simulink model "flexpes_phctrlr_sys"  (R2025b)
settings: Solver=VariableStepAuto  StartTime=0.0  StopTime=1e-6  RelTol=1e-3
values from neighbouring files (symbols this model uses):
  debouncer_cycles = 5    [choPLL_loop_impl.m]
  F_lock_thr = 1    [choPLL_loop_impl.m]
  FPGA_CLK = 125e6    (= 125000000)    [choPLL_loop_impl.m]
  FPGA_Ts = 1./FPGA_CLK    (= 8e-09)    [choPLL_loop_impl.m]
  IIR_C_X = G_loopfilt*my_num_loop_filtZ(1)    [choPLL_loop_impl.m]
  IIR_C_X1 = G_loopfilt*my_num_loop_filtZ(2)    [choPLL_loop_impl.m]
  IIR_C_Y1 = -my_den_loop_filtZ(2)    [choPLL_loop_impl.m]
  max_unwrap_periods = 50    [choPLL_loop_impl.m]
  PFD_CLK = 100e3    (= 100000)    [choPLL_loop_impl.m]
  PFD_Ts = 1./PFD_CLK    (= 1e-05)    [choPLL_loop_impl.m]
  PH_lock_thr = 4    [choPLL_loop_impl.m]
  PHCTRLR_CLK = 100    [choPLL_loop_impl.m]
  PHCTRLR_Ts = 1./PHCTRLR_CLK    (= 0.01)    [choPLL_loop_impl.m]
  TDC_cnt_per_period = round(FPGA_CLK/Fref)    [choPLL_loop_impl.m]
  unwrap_res_period_thr = 0    [choPLL_loop_impl.m]
  unwrap_reset_inhibit_cycles = 20000    [choPLL_loop_impl.m]
  wrap_detect_thr = round(TDC_cnt_per_period*0.55)    [choPLL_loop_impl.m]
libraries: hdlBasic x276, hdlUtilities x4, hdlDSPIP x4, vmcUtilities x1
(part 3 of 3)

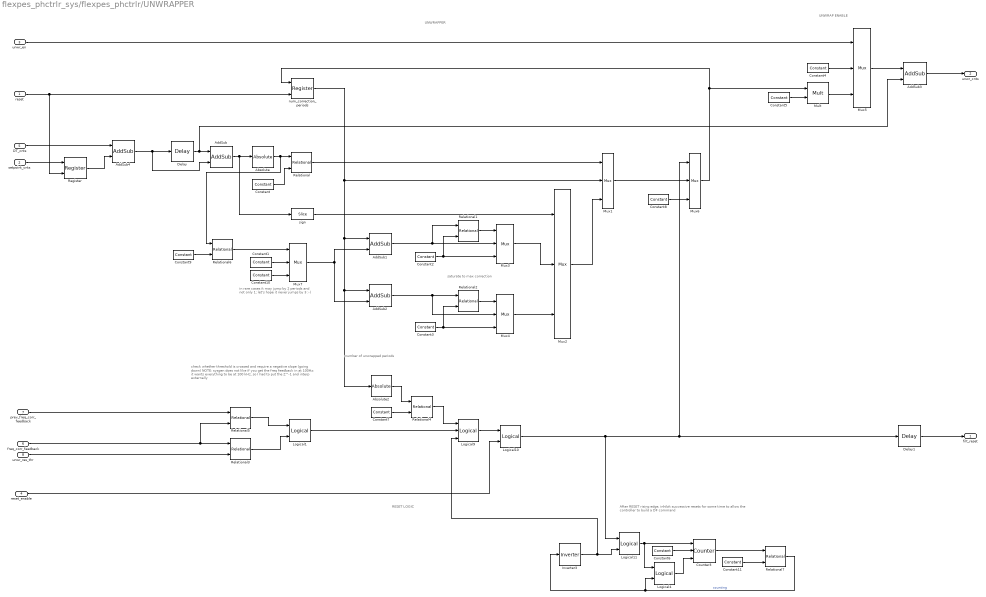
== system flexpes_phctrlr_sys/flexpes_phctrlr/UNWRAPPER ==
  note: UNWRAPPER
  note: saturate to max correction
  note: RESET LOGIC
  note: UNWRAP ENABLE
  note: check whether threshold is crossed and require
      | a negative slope (going down)
      | NOTE: sysgen does not like if you get the freq feedback in
      | at 100Hz: it wants everything to be at 100 kHz, so I had to
      | put the Z^-1 and interp externally
  note: number of unwrapped periods
  note: in rare cases it may jump by 2 periods and not only 1; let's hope it never jumps by 3 :-)
  note: After RESET rising edge, inhibit successive resets for some time
      | to allow the controller to build a DF command
  reset : Inport
  setpoint_cnts : Inport  Port=2
  unwr_en : Inport  Port=3
  reset_enable : Inport  Port=4
  DT_cnts : Inport  Port=5
  freq_corr_feedback : Inport  Port=6
  prev_freq_corr_feedback : Inport  Port=7
  unwr_res_thr : Inport  Port=8
  Absolute : hdlBasic/Absolute  precision=User Defined  arith_type="Signed  (2's comp)"  n_bits=17  bin_pt=0  quantization=Truncate  overflow=Saturate  en=off  latency=0  XmcBlockStatus=1  maskContainerNames=tabcontainer1  block_type=abs  block_config=sysgen:Abs_config
  Absolute2 : hdlBasic/Absolute  precision=User Defined  arith_type="Signed  (2's comp)"  n_bits=17  bin_pt=0  quantization=Truncate  overflow=Saturate  en=off  latency=0  XmcBlockStatus=1  maskContainerNames=tabcontainer1  block_type=abs  block_config=sysgen:Abs_config
  AddSub : hdlBasic/AddSub  mode=Subtraction  use_carryin=off  use_carryout=off  en=off  latency=1  precision=User Defined  arith_type="Signed  (2's comp)"  n_bits=17  bin_pt=0  quantization=Truncate  overflow=Saturate  use_behavioral_HDL=off  hw_selection=Fabric  pipelined=off  XmcBlockStatus=1  maskContainerNames=tabcontainer1  block_type=addsub  block_config=sysgen:Addsub_config
  AddSub1 : hdlBasic/AddSub  mode=Addition  use_carryin=off  use_carryout=off  en=off  latency=0  precision=User Defined  arith_type="Signed  (2's comp)"  n_bits=7  bin_pt=0  quantization=Truncate  overflow=Saturate  use_behavioral_HDL=off  hw_selection=Fabric  pipelined=off  XmcBlockStatus=1  maskContainerNames=tabcontainer1  block_type=addsub  block_config=sysgen:Addsub_config
  AddSub2 : hdlBasic/AddSub  mode=Subtraction  use_carryin=off  use_carryout=off  en=off  latency=0  precision=User Defined  arith_type="Signed  (2's comp)"  n_bits=7  bin_pt=0  quantization=Truncate  overflow=Saturate  use_behavioral_HDL=off  hw_selection=Fabric  pipelined=off  XmcBlockStatus=1  maskContainerNames=tabcontainer1  block_type=addsub  block_config=sysgen:Addsub_config
  AddSub3 : hdlBasic/AddSub  mode=Addition  use_carryin=off  use_carryout=off  en=off  latency=0  precision=User Defined  arith_type="Signed  (2's comp)"  n_bits=17  bin_pt=0  quantization="Round  (unbiased: +/- Inf)"  overflow=Saturate  use_behavioral_HDL=off  hw_selection=Fabric  pipelined=off  XmcBlockStatus=1  maskContainerNames=tabcontainer1  block_type=addsub  block_config=sysgen:Addsub_config
  AddSub4 : hdlBasic/AddSub  mode=Subtraction  use_carryin=off  use_carryout=off  en=off  latency=1  precision=User Defined  arith_type="Signed  (2's comp)"  n_bits=17  bin_pt=0  quantization="Round  (unbiased: +/- Inf)"  overflow=Saturate  use_behavioral_HDL=off  hw_selection=Fabric  pipelined=off  XmcBlockStatus=1  maskContainerNames=tabcontainer1  block_type=addsub  block_config=sysgen:Addsub_config
  Constant : hdlBasic/Constant  const=wrap_detect_thr  gui_display_data_type=Fixed-point  arith_type=Signed (2's comp)  n_bits=17  bin_pt=0  preci_type=Single  exp_width=8  frac_width=24  explicit_period=off  period=1  XmcBlockStatus=1  maskContainerNames=tabcontainer1  block_type=constant  block_config=sysgen:Constant_config
  Constant1 : hdlBasic/Constant  const=1  gui_display_data_type=Fixed-point  arith_type=Signed (2's comp)  n_bits=7  bin_pt=0  preci_type=Single  exp_width=8  frac_width=24  explicit_period=off  period=1  XmcBlockStatus=1  maskContainerNames=tabcontainer1  block_type=constant  block_config=sysgen:Constant_config
  Constant10 : hdlBasic/Constant  const=2  gui_display_data_type=Fixed-point  arith_type=Signed (2's comp)  n_bits=7  bin_pt=0  preci_type=Single  exp_width=8  frac_width=24  explicit_period=off  period=1  XmcBlockStatus=1  maskContainerNames=tabcontainer1  block_type=constant  block_config=sysgen:Constant_config
  Constant11 : hdlBasic/Constant  const=1  gui_display_data_type=Fixed-point  arith_type=Unsigned  n_bits=20  bin_pt=0  preci_type=Single  exp_width=8  frac_width=24  explicit_period=off  period=1  XmcBlockStatus=1  maskContainerNames=tabcontainer1  block_type=constant  block_config=sysgen:Constant_config
  Constant2 : hdlBasic/Constant  const=max_unwrap_periods  gui_display_data_type=Fixed-point  arith_type=Signed (2's comp)  n_bits=7  bin_pt=0  preci_type=Single  exp_width=8  frac_width=24  explicit_period=off  period=1  XmcBlockStatus=1  maskContainerNames=tabcontainer1  block_type=constant  block_config=sysgen:Constant_config
  Constant3 : hdlBasic/Constant  const=-max_unwrap_periods  gui_display_data_type=Fixed-point  arith_type=Signed (2's comp)  n_bits=7  bin_pt=0  preci_type=Single  exp_width=8  frac_width=24  explicit_period=off  period=1  XmcBlockStatus=1  maskContainerNames=tabcontainer1  block_type=constant  block_config=sysgen:Constant_config
  Constant4 : hdlBasic/Constant  const=0  gui_display_data_type=Fixed-point  arith_type=Signed (2's comp)  n_bits=17  bin_pt=0  preci_type=Single  exp_width=8  frac_width=24  explicit_period=off  period=1  XmcBlockStatus=1  maskContainerNames=tabcontainer1  block_type=constant  block_config=sysgen:Constant_config
  Constant5 : hdlBasic/Constant  const=TDC_cnt_per_period  gui_display_data_type=Fixed-point  arith_type=Signed (2's comp)  n_bits=17  bin_pt=0  preci_type=Single  exp_width=8  frac_width=24  explicit_period=off  period=1  XmcBlockStatus=1  maskContainerNames=tabcontainer1  block_type=constant  block_config=sysgen:Constant_config
  Constant6 : hdlBasic/Constant  const=unwrap_reset_inhibit_cycles  gui_display_data_type=Fixed-point  arith_type=Unsigned  n_bits=20  bin_pt=0  preci_type=Single  exp_width=8  frac_width=24  explicit_period=off  period=1  XmcBlockStatus=1  maskContainerNames=tabcontainer1  block_type=constant  block_config=sysgen:Constant_config
  Constant7 : hdlBasic/Constant  const=unwrap_res_period_thr  gui_display_data_type=Fixed-point  arith_type=Signed (2's comp)  n_bits=17  bin_pt=0  preci_type=Single  exp_width=8  frac_width=24  explicit_period=off  period=1  XmcBlockStatus=1  maskContainerNames=tabcontainer1  block_type=constant  block_config=sysgen:Constant_config
  Constant8 : hdlBasic/Constant  const=0  gui_display_data_type=Fixed-point  arith_type=Signed (2's comp)  n_bits=7  bin_pt=0  preci_type=Single  exp_width=8  frac_width=24  explicit_period=off  period=1  XmcBlockStatus=1  maskContainerNames=tabcontainer1  block_type=constant  block_config=sysgen:Constant_config
  Constant9 : hdlBasic/Constant  const=wrap_detect_thr+TDC_cnt_per_period  gui_display_data_type=Fixed-point  arith_type=Signed (2's comp)  n_bits=17  bin_pt=0  preci_type=Single  exp_width=8  frac_width=24  explicit_period=off  period=1  XmcBlockStatus=1  maskContainerNames=tabcontainer1  block_type=constant  block_config=sysgen:Constant_config
  Counter3 : hdlBasic/Counter  cnt_type=Free running  cnt_to=2  operation=Down  start_count=1  cnt_by_val=1  arith_type=Unsigned  n_bits=20  bin_pt=0  load_pin=on  rst=off  en=on  explicit_period=Explicit  period=PFD_Ts  use_behavioral_HDL=off  implementation=Fabric  XmcBlockStatus=1  maskContainerNames=group1  block_type=counter  block_config=sysgen:Counter_config  block_width=531  block_height=1023
  Delay : hdlBasic/Delay  rst=off  en=off  latency=1  reg_retiming=off  XmcBlockStatus=1  maskContainerNames=group1  block_type=delay  block_config=sysgen:Delay_config
  Delay1 : hdlBasic/Delay  rst=off  en=off  latency=1  reg_retiming=off  XmcBlockStatus=1  maskContainerNames=group1  block_type=delay  block_config=sysgen:Delay_config
  Inverter3 : hdlBasic/Inverter  en=off  latency=0  XmcBlockStatus=1  maskContainerNames=group2  block_type=inv  block_config=sysgen:Inverter_config
  Logical1 : hdlBasic/Logical  logical_function=AND  inputs=2  en=off  latency=0  precision=Full  arith_type=Unsigned  n_bits=16  bin_pt=0  align_bp=on  overflow=[]  quantization=[]  XmcBlockStatus=1  maskContainerNames=tabcontainer1  block_type=logical  block_config=sysgen:Logical_config
  Logical10 : hdlBasic/Logical  logical_function=AND  inputs=2  en=off  latency=0  precision=Full  arith_type=Unsigned  n_bits=16  bin_pt=0  align_bp=on  overflow=[]  quantization=[]  XmcBlockStatus=1  maskContainerNames=tabcontainer1  block_type=logical  block_config=sysgen:Logical_config
  Logical11 : hdlBasic/Logical  logical_function=AND  inputs=2  en=off  latency=0  precision=Full  arith_type=Unsigned  n_bits=16  bin_pt=0  align_bp=on  overflow=[]  quantization=[]  XmcBlockStatus=1  maskContainerNames=tabcontainer1  block_type=logical  block_config=sysgen:Logical_config
  Logical4 : hdlBasic/Logical  logical_function=OR  inputs=2  en=off  latency=0  precision=Full  arith_type=Unsigned  n_bits=16  bin_pt=0  align_bp=on  overflow=[]  quantization=[]  XmcBlockStatus=1  maskContainerNames=tabcontainer1  block_type=logical  block_config=sysgen:Logical_config
  Logical9 : hdlBasic/Logical  logical_function=AND  inputs=3  en=off  latency=0  precision=Full  arith_type=Unsigned  n_bits=16  bin_pt=0  align_bp=on  overflow=[]  quantization=[]  XmcBlockStatus=1  maskContainerNames=tabcontainer1  block_type=logical  block_config=sysgen:Logical_config
  Mult : hdlBasic/Mult  precision=User Defined  arith_type="Signed  (2's comp)"  n_bits=17  bin_pt=0  quantization=Truncate  overflow=Saturate  en=off  latency=0  opt_float=off  fp_mult_usage=No Usage  use_behavioral_HDL=off  opt=Speed  use_embedded=on  optimum_pipeline=off  pipeline=on  use_rpm=on  placement_style=Triangular  XmcBlockStatus=1  maskContainerNames=group1  block_type=mult  block_config=sysgen:Mult_config  block_width=598  block_height=876
  Mux{1..7} (7 alike) : hdlBasic/Mux  inputs=2  en=off  latency=0  precision=Full  arith_type=Unsigned  n_bits=16  bin_pt=14  quantization=Truncate  overflow=Wrap  XmcBlockStatus=1  maskContainerNames=tabcontainer1  block_type=mux  block_config=sysgen:Mux_config
  Register : hdlBasic/Register  init=0  rst=on  en=off  XmcBlockStatus=1  maskContainerNames=tabcontainer1  block_type=register  block_config=sysgen:Register_config
  Relational{,1,5..6} (4 alike) : hdlBasic/Relational  mode=a>=b  op_type=Bool  en=off  latency=0  XmcBlockStatus=1  maskContainerNames=tabcontainer1  block_type=relational  block_config=sysgen:Relational_config
  Relational2 : hdlBasic/Relational  mode=a<=b  op_type=Bool  en=off  latency=0  XmcBlockStatus=1  maskContainerNames=tabcontainer1  block_type=relational  block_config=sysgen:Relational_config
  Relational3 : hdlBasic/Relational  mode=a<b  op_type=Bool  en=off  latency=0  XmcBlockStatus=1  maskContainerNames=tabcontainer1  block_type=relational  block_config=sysgen:Relational_config
  Relational4 : hdlBasic/Relational  mode=a>b  op_type=Bool  en=off  latency=0  XmcBlockStatus=1  maskContainerNames=tabcontainer1  block_type=relational  block_config=sysgen:Relational_config
  Relational7 : hdlBasic/Relational  mode=a!=b  op_type=Bool  en=off  latency=0  XmcBlockStatus=1  maskContainerNames=tabcontainer1  block_type=relational  block_config=sysgen:Relational_config
  num_correction_periods : hdlBasic/Register  init=0  rst=on  en=off  XmcBlockStatus=1  maskContainerNames=tabcontainer1  block_type=register  block_config=sysgen:Register_config
  sign : hdlBasic/Slice  nbits=1  boolean_output=on  mode=Upper Bit Location + Width  bit1=0  base1=MSB of Input  bit0=0  base0=LSB of Input  XmcBlockStatus=1  maskContainerNames=group1  block_type=slice  block_config=sysgen:Slice_config
  filt_reset : Outport
  unwr_cnts : Outport  Port=2
  wires:
  Constant2/1 -> Relational1/2, Mux3/3
  sign/1 -> Mux2/1
  AddSub2/1 -> Mux4/2, Relational2/1
  Delay/1 -> AddSub3/2, AddSub/1
  Relational4/1 -> Logical9/1
  num_correction_periods/1 -> AddSub1/1, Absolute2/1, AddSub2/1, Mux1/2
  AddSub1/1 -> Mux3/2, Relational1/1
  reset/1 -> num_correction_periods/2, Register/2
  Constant/1 -> Relational/2
  Relational2/1 -> Mux4/1
  Mult/1 -> Mux5/3
  Relational/1 -> Mux1/1
  AddSub/1 -> sign/1, Absolute/1
  freq_corr_feedback/1 -> Relational5/2, Relational3/1
  Mux2/1 -> Mux1/3
  Mux4/1 -> Mux2/3
  AddSub3/1 -> unwr_cnts/1
  Constant4/1 -> Mux5/2
  Logical9/1 -> Logical10/1
  Mux3/1 -> Mux2/2
  Absolute/1 -> Relational6/1, Relational/1
  Relational1/1 -> Mux3/1
  Mux5/1 -> AddSub3/1
  Constant3/1 -> Relational2/2, Mux4/3
  DT_cnts/1 -> AddSub4/1
  Constant8/1 -> Mux6/3
  Constant7/1 -> Relational4/2
  Absolute2/1 -> Relational4/1
  Constant5/1 -> Mult/2
  Mux1/1 -> Mux6/2
  unwr_en/1 -> Mux5/1
  reset_enable/1 -> Logical10/2
  Delay1/1 -> filt_reset/1
  setpoint_cnts/1 -> Register/1
  unwr_res_thr/1 -> Relational3/2
  prev_freq_corr_feedback/1 -> Relational5/1
  Relational5/1 -> Logical1/1
  Relational3/1 -> Logical1/2
  Logical1/1 -> Logical9/2
  Constant9/1 -> Relational6/2
  Relational6/1 -> Mux7/1
  Mux7/1 -> AddSub2/2, AddSub1/2
  Constant1/1 -> Mux7/2
  Constant10/1 -> Mux7/3
  AddSub4/1 -> AddSub/2, Delay/1
  Register/1 -> AddSub4/2
  Logical4/1 -> Counter3/3
  Logical10/1 -> Logical11/1, Delay1/1, Mux6/1
  Counter3/1 -> Relational7/1
  Constant6/1 -> Counter3/2
  Inverter3/1 -> Logical9/3, Logical11/2
  Logical11/1 -> Logical4/1, Counter3/1
  Constant11/1 -> Relational7/2
  Relational7/1 -> Inverter3/1, Logical4/2  "counting"
  Mux6/1 -> num_correction_periods/1, Mult/1
